simulink model "watertanksystem"  (R2023a)
settings: Solver=VariableStepAuto  StartTime=0.0  StopTime=1000  RelTol=1e-3
values from neighbouring files (symbols this model uses):
  R = 400    [parameter.m]
  S = (D/2)^2*pi    (= 0.196349540849)    [parameter.m]
settings Model: Creator=mosuk  LastModifiedBy=mosuk

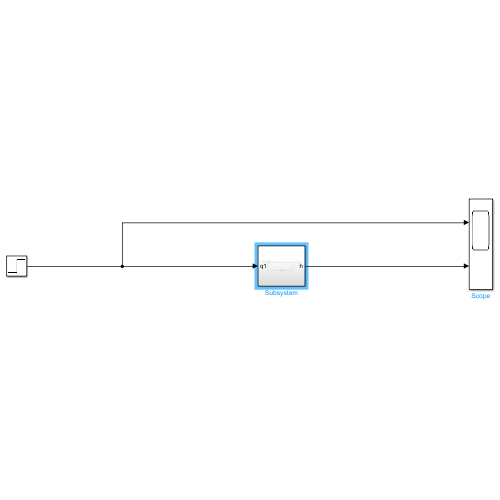
[thumbnail: Simulink's stored preview of the top-level diagram]
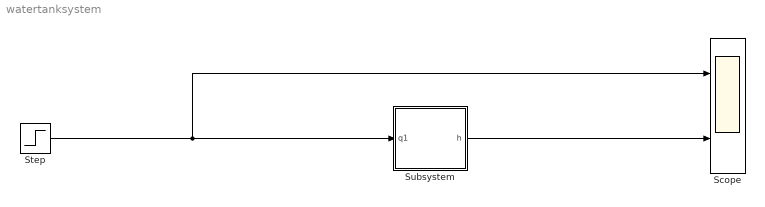
== system watertanksystem ==
  Scope : Scope  NumInputPorts=2
  Step : Step  SampleTime=0
  Subsystem : Subsystem
  wires:
  Step/1 -> Scope/1, Subsystem/1(q1)
  Subsystem/1(h) -> Scope/2

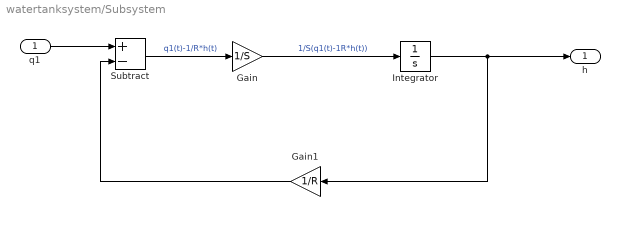
== system watertanksystem/Subsystem ==
  q1 : Inport
  Gain : Gain  Gain=1/S
  Gain1 : Gain  Gain=1/R
  Integrator : Integrator
  Subtract : Sum  Inputs=+-
  h : Outport
  wires:
  Integrator/1 -> h/1, Gain1/1
  Gain/1 -> Integrator/1  "1/S(q1(t)-1R*h(t))"
  q1/1 -> Subtract/1
  Subtract/1 -> Gain/1  "q1(t)-1/R*h(t)"
  Gain1/1 -> Subtract/2
